simulink model "test_mdl_NI"  (R2018a)
settings: Solver=VariableStepAuto  StartTime=0.0  StopTime=10.0  RelTol=1e-3
(part 12 of 24)

== system test_mdl_NI/Subsystem/IPMA_ADAS/Side_Detect_L_Stat_Ox3A6 ==
  in_port : Inport
  BttLeft_D_RqDrv : Terminator
  BttLeft_D_Stat : Terminator
  CtaAlrtLeft2_D_Stat : Terminator
  CtaAlrtLeft_D_Stat : Terminator
  CtaBrkLeftMsgTxt_B_Rq : Terminator
  CtaLeftBrkDecel_B_Rq : Terminator
  CtaLeftBrkEnbl_B_Rq : Terminator
  CtaLeft_D_Stat : Terminator
  CtaSnsLeft_D_Stat : Terminator
  Side_Detect_L_Illum : Terminator
  SodAlrtLeft_D_Stat : Terminator
  SodDetctLeft_D_Stat : Terminator
  SodLeft_D_Stat : Terminator
  SodSnsLeft_D_Stat : Terminator
  SodWarnLeft_Prd_Rq : Terminator
  bus_selector : BusSelector  OutputSignals=BttLeft_D_RqDrv,BttLeft_D_Stat,CtaAlrtLeft2_D_Stat,CtaAlrtLeft_D_Stat,CtaBrkLeftMsgTxt_B_Rq,CtaLeftBrkDecel_B_Rq,CtaLeftBrkEnbl_B_Rq,CtaLeft_D_Stat,CtaSnsLeft_D_Stat,Side_Detect_L_Illum,SodAlrtLeft_D_Stat,SodDetctLeft_D_Stat,SodLeft_D_Stat,SodSnsLeft_D_Stat,SodWarnLeft_Prd_Rq
  wires:
  in_port/1 -> bus_selector/1  "Side_Detect_L_Stat_Ox3A6"
  bus_selector/1 -> BttLeft_D_RqDrv/1  "<BttLeft_D_RqDrv>"
  bus_selector/2 -> BttLeft_D_Stat/1  "<BttLeft_D_Stat>"
  bus_selector/3 -> CtaAlrtLeft2_D_Stat/1  "<CtaAlrtLeft2_D_Stat>"
  bus_selector/4 -> CtaAlrtLeft_D_Stat/1  "<CtaAlrtLeft_D_Stat>"
  bus_selector/5 -> CtaBrkLeftMsgTxt_B_Rq/1  "<CtaBrkLeftMsgTxt_B_Rq>"
  bus_selector/6 -> CtaLeftBrkDecel_B_Rq/1  "<CtaLeftBrkDecel_B_Rq>"
  bus_selector/7 -> CtaLeftBrkEnbl_B_Rq/1  "<CtaLeftBrkEnbl_B_Rq>"
  bus_selector/8 -> CtaLeft_D_Stat/1  "<CtaLeft_D_Stat>"
  bus_selector/9 -> CtaSnsLeft_D_Stat/1  "<CtaSnsLeft_D_Stat>"
  bus_selector/10 -> Side_Detect_L_Illum/1  "<Side_Detect_L_Illum>"
  bus_selector/11 -> SodAlrtLeft_D_Stat/1  "<SodAlrtLeft_D_Stat>"
  bus_selector/12 -> SodDetctLeft_D_Stat/1  "<SodDetctLeft_D_Stat>"
  bus_selector/13 -> SodLeft_D_Stat/1  "<SodLeft_D_Stat>"
  bus_selector/14 -> SodSnsLeft_D_Stat/1  "<SodSnsLeft_D_Stat>"
  bus_selector/15 -> SodWarnLeft_Prd_Rq/1  "<SodWarnLeft_Prd_Rq>"

== system test_mdl_NI/Subsystem/IPMA_ADAS/Side_Detect_R_Stat_Ox3A7 ==
  in_port : Inport
  BttRight_D_RqDrv : Terminator
  BttRight_D_Stat : Terminator
  CtaAlrtRight2_D_Stat : Terminator
  CtaAlrtRight_D_Stat : Terminator
  CtaBrkRightMsgTxt_B_Rq : Terminator
  CtaRightBrkDecel_B_Rq : Terminator
  CtaRightBrkEnbl_B_Rq : Terminator
  CtaRight_D_Stat : Terminator
  CtaSnsRight_D_Stat : Terminator
  Side_Detect_R_Illum : Terminator
  SodAlrtRight_D_Stat : Terminator
  SodDetctRight_D_Stat : Terminator
  SodRight_D_Stat : Terminator
  SodSnsRight_D_Stat : Terminator
  SodWarnRight_Prd_Rq : Terminator
  bus_selector : BusSelector  OutputSignals=BttRight_D_RqDrv,BttRight_D_Stat,CtaAlrtRight2_D_Stat,CtaAlrtRight_D_Stat,CtaBrkRightMsgTxt_B_Rq,CtaRightBrkDecel_B_Rq,CtaRightBrkEnbl_B_Rq,CtaRight_D_Stat,CtaSnsRight_D_Stat,Side_Detect_R_Illum,SodAlrtRight_D_Stat,SodDetctRight_D_Stat,SodRight_D_Stat,SodSnsRight_D_Stat,SodWarnRight_Prd_Rq
  wires:
  in_port/1 -> bus_selector/1  "Side_Detect_R_Stat_Ox3A7"
  bus_selector/1 -> BttRight_D_RqDrv/1  "<BttRight_D_RqDrv>"
  bus_selector/2 -> BttRight_D_Stat/1  "<BttRight_D_Stat>"
  bus_selector/3 -> CtaAlrtRight2_D_Stat/1  "<CtaAlrtRight2_D_Stat>"
  bus_selector/4 -> CtaAlrtRight_D_Stat/1  "<CtaAlrtRight_D_Stat>"
  bus_selector/5 -> CtaBrkRightMsgTxt_B_Rq/1  "<CtaBrkRightMsgTxt_B_Rq>"
  bus_selector/6 -> CtaRightBrkDecel_B_Rq/1  "<CtaRightBrkDecel_B_Rq>"
  bus_selector/7 -> CtaRightBrkEnbl_B_Rq/1  "<CtaRightBrkEnbl_B_Rq>"
  bus_selector/8 -> CtaRight_D_Stat/1  "<CtaRight_D_Stat>"
  bus_selector/9 -> CtaSnsRight_D_Stat/1  "<CtaSnsRight_D_Stat>"
  bus_selector/10 -> Side_Detect_R_Illum/1  "<Side_Detect_R_Illum>"
  bus_selector/11 -> SodAlrtRight_D_Stat/1  "<SodAlrtRight_D_Stat>"
  bus_selector/12 -> SodDetctRight_D_Stat/1  "<SodDetctRight_D_Stat>"
  bus_selector/13 -> SodRight_D_Stat/1  "<SodRight_D_Stat>"
  bus_selector/14 -> SodSnsRight_D_Stat/1  "<SodSnsRight_D_Stat>"
  bus_selector/15 -> SodWarnRight_Prd_Rq/1  "<SodWarnRight_Prd_Rq>"

== system test_mdl_NI/Subsystem/IPMA_ADAS/Steer_Assist_Data_Ox3D7 ==
  in_port : Inport
  CmbbObjClass_D_Stat : Terminator
  CmbbObjColl_T_Actl : Terminator
  CmbbObjConfdnc_D_Stat : Terminator
  CmbbObjDistLat_L_Actl : Terminator
  CmbbObjDistLong_L_Actl : Terminator
  CmbbObjRelLat_V_Actl : Terminator
  CmbbObjRelLong_V_Actl : Terminator
  EsaEnbl_D2_Rq : Terminator
  bus_selector : BusSelector  OutputSignals=CmbbObjClass_D_Stat,CmbbObjColl_T_Actl,CmbbObjConfdnc_D_Stat,CmbbObjDistLat_L_Actl,CmbbObjDistLong_L_Actl,CmbbObjRelLat_V_Actl,CmbbObjRelLong_V_Actl,EsaEnbl_D2_Rq
  wires:
  in_port/1 -> bus_selector/1  "Steer_Assist_Data_Ox3D7"
  bus_selector/1 -> CmbbObjClass_D_Stat/1  "<CmbbObjClass_D_Stat>"
  bus_selector/2 -> CmbbObjColl_T_Actl/1  "<CmbbObjColl_T_Actl>"
  bus_selector/3 -> CmbbObjConfdnc_D_Stat/1  "<CmbbObjConfdnc_D_Stat>"
  bus_selector/4 -> CmbbObjDistLat_L_Actl/1  "<CmbbObjDistLat_L_Actl>"
  bus_selector/5 -> CmbbObjDistLong_L_Actl/1  "<CmbbObjDistLong_L_Actl>"
  bus_selector/6 -> CmbbObjRelLat_V_Actl/1  "<CmbbObjRelLat_V_Actl>"
  bus_selector/7 -> CmbbObjRelLong_V_Actl/1  "<CmbbObjRelLong_V_Actl>"
  bus_selector/8 -> EsaEnbl_D2_Rq/1  "<EsaEnbl_D2_Rq>"

== system test_mdl_NI/Subsystem/IPMA_ADAS/SuspensionRoad_Data_Ox3D0 ==
  in_port : Inport
  SrpDistLeft_L_Actl : Terminator
  SrpDistRight_L_Actl : Terminator
  SrpEventLeft_D_Stat : Terminator
  SrpEventRight_D_Stat : Terminator
  SrpHghtLeft_L_Actl : Terminator
  SrpHghtRight_L_Actl : Terminator
  SrpSigValid_B_Stat : Terminator
  SuspClkSync_No_Actl : Terminator
  bus_selector : BusSelector  OutputSignals=SrpDistLeft_L_Actl,SrpDistRight_L_Actl,SrpEventLeft_D_Stat,SrpEventRight_D_Stat,SrpHghtLeft_L_Actl,SrpHghtRight_L_Actl,SrpSigValid_B_Stat,SuspClkSync_No_Actl
  wires:
  in_port/1 -> bus_selector/1  "SuspensionRoad_Data_Ox3D0"
  bus_selector/1 -> SrpDistLeft_L_Actl/1  "<SrpDistLeft_L_Actl>"
  bus_selector/2 -> SrpDistRight_L_Actl/1  "<SrpDistRight_L_Actl>"
  bus_selector/3 -> SrpEventLeft_D_Stat/1  "<SrpEventLeft_D_Stat>"
  bus_selector/4 -> SrpEventRight_D_Stat/1  "<SrpEventRight_D_Stat>"
  bus_selector/5 -> SrpHghtLeft_L_Actl/1  "<SrpHghtLeft_L_Actl>"
  bus_selector/6 -> SrpHghtRight_L_Actl/1  "<SrpHghtRight_L_Actl>"
  bus_selector/7 -> SrpSigValid_B_Stat/1  "<SrpSigValid_B_Stat>"
  bus_selector/8 -> SuspClkSync_No_Actl/1  "<SuspClkSync_No_Actl>"

== system test_mdl_NI/Subsystem/IPMA_ADAS/TesterPhysicalResCCM_Ox76C ==
  in_port : Inport
  TesterPhysicalResCCM : Terminator
  bus_selector : BusSelector  OutputSignals=TesterPhysicalResCCM
  wires:
  in_port/1 -> bus_selector/1  "TesterPhysicalResCCM_Ox76C"
  bus_selector/1 -> TesterPhysicalResCCM/1  "<TesterPhysicalResCCM>"

== system test_mdl_NI/Subsystem/IPMA_ADAS/TesterPhysicalResIPMA_Ox70E ==
  in_port : Inport
  TesterPhysicalResIPMA : Terminator
  bus_selector : BusSelector  OutputSignals=TesterPhysicalResIPMA
  wires:
  in_port/1 -> bus_selector/1  "TesterPhysicalResIPMA_Ox70E"
  bus_selector/1 -> TesterPhysicalResIPMA/1  "<TesterPhysicalResIPMA>"

== system test_mdl_NI/Subsystem/IPMA_ADAS/TesterPhysicalResSODCMC_Ox6FA ==
  in_port : Inport
  TesterPhysicalResSODCMC : Terminator
  bus_selector : BusSelector  OutputSignals=TesterPhysicalResSODCMC
  wires:
  in_port/1 -> bus_selector/1  "TesterPhysicalResSODCMC_Ox6FA"
  bus_selector/1 -> TesterPhysicalResSODCMC/1  "<TesterPhysicalResSODCMC>"

== system test_mdl_NI/Subsystem/IPMA_ADAS/TesterPhysicalResSODCMD_Ox6FB ==
  in_port : Inport
  TesterPhysicalResSODCMD : Terminator
  bus_selector : BusSelector  OutputSignals=TesterPhysicalResSODCMD
  wires:
  in_port/1 -> bus_selector/1  "TesterPhysicalResSODCMD_Ox6FB"
  bus_selector/1 -> TesterPhysicalResSODCMD/1  "<TesterPhysicalResSODCMD>"

== system test_mdl_NI/Subsystem/IPMA_ADAS/TesterPhysicalResSODL_Ox7CC ==
  in_port : Inport
  TesterPhysicalResSODL : Terminator
  bus_selector : BusSelector  OutputSignals=TesterPhysicalResSODL
  wires:
  in_port/1 -> bus_selector/1  "TesterPhysicalResSODL_Ox7CC"
  bus_selector/1 -> TesterPhysicalResSODL/1  "<TesterPhysicalResSODL>"

== system test_mdl_NI/Subsystem/IPMA_ADAS/TesterPhysicalResSODR_Ox7CE ==
  in_port : Inport
  TesterPhysicalResSODR : Terminator
  bus_selector : BusSelector  OutputSignals=TesterPhysicalResSODR
  wires:
  in_port/1 -> bus_selector/1  "TesterPhysicalResSODR_Ox7CE"
  bus_selector/1 -> TesterPhysicalResSODR/1  "<TesterPhysicalResSODR>"

== system test_mdl_NI/Subsystem/IPMA_ADAS/Traffic_RecognitnData_Ox3CD ==
  in_port : Inport
  TsrMsgTxt_D_Rq : Terminator
  TsrOswWarnMsgTxt_D_Rq : Terminator
  TsrOvtkMsgTxt2_D_Rq : Terminator
  TsrOvtkMsgTxt_D_Rq : Terminator
  TsrOvtkStatMsgTxt_D_Rq : Terminator
  TsrStatMsgTxt_D_Rq : Terminator
  TsrVLim1MsgTxt_D_Rq : Terminator
  TsrVLim2MsgTxt_D_Rq : Terminator
  TsrVl1PrmntMsgTxt_D_Rq : Terminator
  TsrVl1RstrcMsgTxt2_D_Rq : Terminator
  TsrVl1RstrcMsgTxt_D_Rq : Terminator
  TsrVl1StatMsgTxt_D_Rq : Terminator
  TsrVl2PrmntMsgTxt_D_Rq : Terminator
  TsrVl2RstrcMsgTxt2_D_Rq : Terminator
  TsrVl2RstrcMsgTxt_D_Rq : Terminator
  TsrVl2StatMsgTxt_D_Rq : Terminator
  TsrVlUnitMsgTxt_D_Rq : Terminator
  WwaWarn_B_Rq : Terminator
  bus_selector : BusSelector  OutputSignals=TsrMsgTxt_D_Rq,TsrOswWarnMsgTxt_D_Rq,TsrOvtkMsgTxt2_D_Rq,TsrOvtkMsgTxt_D_Rq,TsrOvtkStatMsgTxt_D_Rq,TsrStatMsgTxt_D_Rq,TsrVLim1MsgTxt_D_Rq,TsrVLim2MsgTxt_D_Rq,TsrVl1PrmntMsgTxt_D_Rq,TsrVl1RstrcMsgTxt2_D_Rq,TsrVl1RstrcMsgTxt_D_Rq,TsrVl1StatMsgTxt_D_Rq,TsrVl2PrmntMsgTxt_D_Rq,TsrVl2RstrcMsgTxt2_D_Rq,TsrVl2RstrcMsgTxt_D_Rq,TsrVl2StatMsgTxt_D_Rq,TsrVlUnitMsgTxt_D_Rq,WwaWarn_B_Rq
  wires:
  in_port/1 -> bus_selector/1  "Traffic_RecognitnData_Ox3CD"
  bus_selector/1 -> TsrMsgTxt_D_Rq/1  "<TsrMsgTxt_D_Rq>"
  bus_selector/2 -> TsrOswWarnMsgTxt_D_Rq/1  "<TsrOswWarnMsgTxt_D_Rq>"
  bus_selector/3 -> TsrOvtkMsgTxt2_D_Rq/1  "<TsrOvtkMsgTxt2_D_Rq>"
  bus_selector/4 -> TsrOvtkMsgTxt_D_Rq/1  "<TsrOvtkMsgTxt_D_Rq>"
  bus_selector/5 -> TsrOvtkStatMsgTxt_D_Rq/1  "<TsrOvtkStatMsgTxt_D_Rq>"
  bus_selector/6 -> TsrStatMsgTxt_D_Rq/1  "<TsrStatMsgTxt_D_Rq>"
  bus_selector/7 -> TsrVLim1MsgTxt_D_Rq/1  "<TsrVLim1MsgTxt_D_Rq>"
  bus_selector/8 -> TsrVLim2MsgTxt_D_Rq/1  "<TsrVLim2MsgTxt_D_Rq>"
  bus_selector/9 -> TsrVl1PrmntMsgTxt_D_Rq/1  "<TsrVl1PrmntMsgTxt_D_Rq>"
  bus_selector/10 -> TsrVl1RstrcMsgTxt2_D_Rq/1  "<TsrVl1RstrcMsgTxt2_D_Rq>"
  bus_selector/11 -> TsrVl1RstrcMsgTxt_D_Rq/1  "<TsrVl1RstrcMsgTxt_D_Rq>"
  bus_selector/12 -> TsrVl1StatMsgTxt_D_Rq/1  "<TsrVl1StatMsgTxt_D_Rq>"
  bus_selector/13 -> TsrVl2PrmntMsgTxt_D_Rq/1  "<TsrVl2PrmntMsgTxt_D_Rq>"
  bus_selector/14 -> TsrVl2RstrcMsgTxt2_D_Rq/1  "<TsrVl2RstrcMsgTxt2_D_Rq>"
  bus_selector/15 -> TsrVl2RstrcMsgTxt_D_Rq/1  "<TsrVl2RstrcMsgTxt_D_Rq>"
  bus_selector/16 -> TsrVl2StatMsgTxt_D_Rq/1  "<TsrVl2StatMsgTxt_D_Rq>"
  bus_selector/17 -> TsrVlUnitMsgTxt_D_Rq/1  "<TsrVlUnitMsgTxt_D_Rq>"
  bus_selector/18 -> WwaWarn_B_Rq/1  "<WwaWarn_B_Rq>"

== system test_mdl_NI/Subsystem/IPMA_ADAS/TrailerAid_Stat3_Ox459 ==
  in_port : Inport
  HitchToTrlrAxle_L_Calc2 : Terminator
  HitchToVehAxle_L_Calc : Terminator
  TrlrAidTrgtId_No_Actl : Terminator
  TrlrAid_An3_Actl : Terminator
  TrlrAid_AnRate2_Actl : Terminator
  TrlrAid_D2_Stat : Terminator
  TrlrAnCalib_B_Complt : Terminator
  TrlrAnOffstDir_D_Calc : Terminator
  TrlrAnOffst_An_Calc : Terminator
  TrlrRvrse_D_Stat : Terminator
  TrlrTrgtAcquire_D_Stat : Terminator
  bus_selector : BusSelector  OutputSignals=HitchToTrlrAxle_L_Calc2,HitchToVehAxle_L_Calc,TrlrAidTrgtId_No_Actl,TrlrAid_An3_Actl,TrlrAid_AnRate2_Actl,TrlrAid_D2_Stat,TrlrAnCalib_B_Complt,TrlrAnOffstDir_D_Calc,TrlrAnOffst_An_Calc,TrlrRvrse_D_Stat,TrlrTrgtAcquire_D_Stat
  wires:
  in_port/1 -> bus_selector/1  "TrailerAid_Stat3_Ox459"
  bus_selector/1 -> HitchToTrlrAxle_L_Calc2/1  "<HitchToTrlrAxle_L_Calc2>"
  bus_selector/2 -> HitchToVehAxle_L_Calc/1  "<HitchToVehAxle_L_Calc>"
  bus_selector/3 -> TrlrAidTrgtId_No_Actl/1  "<TrlrAidTrgtId_No_Actl>"
  bus_selector/4 -> TrlrAid_An3_Actl/1  "<TrlrAid_An3_Actl>"
  bus_selector/5 -> TrlrAid_AnRate2_Actl/1  "<TrlrAid_AnRate2_Actl>"
  bus_selector/6 -> TrlrAid_D2_Stat/1  "<TrlrAid_D2_Stat>"
  bus_selector/7 -> TrlrAnCalib_B_Complt/1  "<TrlrAnCalib_B_Complt>"
  bus_selector/8 -> TrlrAnOffstDir_D_Calc/1  "<TrlrAnOffstDir_D_Calc>"
  bus_selector/9 -> TrlrAnOffst_An_Calc/1  "<TrlrAnOffst_An_Calc>"
  bus_selector/10 -> TrlrRvrse_D_Stat/1  "<TrlrRvrse_D_Stat>"
  bus_selector/11 -> TrlrTrgtAcquire_D_Stat/1  "<TrlrTrgtAcquire_D_Stat>"

== system test_mdl_NI/Subsystem/PCM/DCACA_Data4_Ox36E ==
  in_port : Inport
  DcacElPw_D_Stat : Terminator
  DcacEngOnMsgTxt_D_Rq : Terminator
  DcacFaltMsgTxt_D_Rq : Terminator
  DcacGfciTest_B_Rq : Terminator
  DcacHw_D_Confg : Terminator
  DcacLedCtl_D_Rq : Terminator
  DcacLoFuelMsgTxt_D_Rq : Terminator
  DcacOn_B_Rq : Terminator
  DcacOut1_Pw_Dsply : Terminator
  DcacOut2_Pw_Dsply : Terminator
  DcacOut_Pw_DsplyMx : Terminator
  DcacSys_B_Falt : Terminator
  PwBedPnlEnbl_B_Rq : Terminator
  bus_selector : BusSelector  OutputSignals=DcacElPw_D_Stat,DcacEngOnMsgTxt_D_Rq,DcacFaltMsgTxt_D_Rq,DcacGfciTest_B_Rq,DcacHw_D_Confg,DcacLedCtl_D_Rq,DcacLoFuelMsgTxt_D_Rq,DcacOn_B_Rq,DcacOut1_Pw_Dsply,DcacOut2_Pw_Dsply,DcacOut_Pw_DsplyMx,DcacSys_B_Falt,PwBedPnlEnbl_B_Rq
  wires:
  in_port/1 -> bus_selector/1  "DCACA_Data4_Ox36E"
  bus_selector/1 -> DcacElPw_D_Stat/1  "<DcacElPw_D_Stat>"
  bus_selector/2 -> DcacEngOnMsgTxt_D_Rq/1  "<DcacEngOnMsgTxt_D_Rq>"
  bus_selector/3 -> DcacFaltMsgTxt_D_Rq/1  "<DcacFaltMsgTxt_D_Rq>"
  bus_selector/4 -> DcacGfciTest_B_Rq/1  "<DcacGfciTest_B_Rq>"
  bus_selector/5 -> DcacHw_D_Confg/1  "<DcacHw_D_Confg>"
  bus_selector/6 -> DcacLedCtl_D_Rq/1  "<DcacLedCtl_D_Rq>"
  bus_selector/7 -> DcacLoFuelMsgTxt_D_Rq/1  "<DcacLoFuelMsgTxt_D_Rq>"
  bus_selector/8 -> DcacOn_B_Rq/1  "<DcacOn_B_Rq>"
  bus_selector/9 -> DcacOut1_Pw_Dsply/1  "<DcacOut1_Pw_Dsply>"
  bus_selector/10 -> DcacOut2_Pw_Dsply/1  "<DcacOut2_Pw_Dsply>"
  bus_selector/11 -> DcacOut_Pw_DsplyMx/1  "<DcacOut_Pw_DsplyMx>"
  bus_selector/12 -> DcacSys_B_Falt/1  "<DcacSys_B_Falt>"
  bus_selector/13 -> PwBedPnlEnbl_B_Rq/1  "<PwBedPnlEnbl_B_Rq>"

== system test_mdl_NI/Subsystem/PCM/EngBrakeData_Ox165 ==
  in_port : Inport
  AccEngStat_D_Actl : Terminator
  AccStopMde_D_Rq : Terminator
  BPedDrvAppl_D_QF : Terminator
  BpedDrvAppl_D_Actl : Terminator
  CcMde_D_Actl : Terminator
  CcOvrrdActv_B_Actl : Terminator
  CcStat_D_Actl : Terminator
  CmbbDeny_B_ActlPrpl : Terminator
  CmbbEngTqMn_B_Actl : Terminator
  EngAout_N_MnAllw : Terminator
  PrplTqMnSat_B_Actl : Terminator
  Veh_V_DsplyCcSet : Terminator
  bus_selector : BusSelector  OutputSignals=AccEngStat_D_Actl,AccStopMde_D_Rq,BPedDrvAppl_D_QF,BpedDrvAppl_D_Actl,CcMde_D_Actl,CcOvrrdActv_B_Actl,CcStat_D_Actl,CmbbDeny_B_ActlPrpl,CmbbEngTqMn_B_Actl,EngAout_N_MnAllw,PrplTqMnSat_B_Actl,Veh_V_DsplyCcSet
  wires:
  in_port/1 -> bus_selector/1  "EngBrakeData_Ox165"
  bus_selector/1 -> AccEngStat_D_Actl/1  "<AccEngStat_D_Actl>"
  bus_selector/2 -> AccStopMde_D_Rq/1  "<AccStopMde_D_Rq>"
  bus_selector/3 -> BPedDrvAppl_D_QF/1  "<BPedDrvAppl_D_QF>"
  bus_selector/4 -> BpedDrvAppl_D_Actl/1  "<BpedDrvAppl_D_Actl>"
  bus_selector/5 -> CcMde_D_Actl/1  "<CcMde_D_Actl>"
  bus_selector/6 -> CcOvrrdActv_B_Actl/1  "<CcOvrrdActv_B_Actl>"
  bus_selector/7 -> CcStat_D_Actl/1  "<CcStat_D_Actl>"
  bus_selector/8 -> CmbbDeny_B_ActlPrpl/1  "<CmbbDeny_B_ActlPrpl>"
  bus_selector/9 -> CmbbEngTqMn_B_Actl/1  "<CmbbEngTqMn_B_Actl>"
  bus_selector/10 -> EngAout_N_MnAllw/1  "<EngAout_N_MnAllw>"
  bus_selector/11 -> PrplTqMnSat_B_Actl/1  "<PrplTqMnSat_B_Actl>"
  bus_selector/12 -> Veh_V_DsplyCcSet/1  "<Veh_V_DsplyCcSet>"

== system test_mdl_NI/Subsystem/PCM/EngVehicleSpThrottle2_Ox202 ==
  in_port : Inport
  GearRvrse_D_Actl : Terminator
  StrtrMtrCtlMsgTxt_D2_Rq : Terminator
  StrtrMtrCtlMsgTxt_D_Rq : Terminator
  StrtrMtrDlyStrt_B_Stat : Terminator
  VehVActlEng_D_Qf : Terminator
  VehVActlEng_No_Cnt : Terminator
  VehVActlEng_No_Cs : Terminator
  VehVTrlrAid_B_Avail : Terminator
  Veh_V_ActlEng : Terminator
  Veh_V_RqCcSet : Terminator
  bus_selector : BusSelector  OutputSignals=GearRvrse_D_Actl,StrtrMtrCtlMsgTxt_D2_Rq,StrtrMtrCtlMsgTxt_D_Rq,StrtrMtrDlyStrt_B_Stat,VehVActlEng_D_Qf,VehVActlEng_No_Cnt,VehVActlEng_No_Cs,VehVTrlrAid_B_Avail,Veh_V_ActlEng,Veh_V_RqCcSet
  wires:
  in_port/1 -> bus_selector/1  "EngVehicleSpThrottle2_Ox202"
  bus_selector/1 -> GearRvrse_D_Actl/1  "<GearRvrse_D_Actl>"
  bus_selector/2 -> StrtrMtrCtlMsgTxt_D2_Rq/1  "<StrtrMtrCtlMsgTxt_D2_Rq>"
  bus_selector/3 -> StrtrMtrCtlMsgTxt_D_Rq/1  "<StrtrMtrCtlMsgTxt_D_Rq>"
  bus_selector/4 -> StrtrMtrDlyStrt_B_Stat/1  "<StrtrMtrDlyStrt_B_Stat>"
  bus_selector/5 -> VehVActlEng_D_Qf/1  "<VehVActlEng_D_Qf>"
  bus_selector/6 -> VehVActlEng_No_Cnt/1  "<VehVActlEng_No_Cnt>"
  bus_selector/7 -> VehVActlEng_No_Cs/1  "<VehVActlEng_No_Cs>"
  bus_selector/8 -> VehVTrlrAid_B_Avail/1  "<VehVTrlrAid_B_Avail>"
  bus_selector/9 -> Veh_V_ActlEng/1  "<Veh_V_ActlEng>"
  bus_selector/10 -> Veh_V_RqCcSet/1  "<Veh_V_RqCcSet>"

== system test_mdl_NI/Subsystem/PCM/EngVehicleSpThrottle_Ox204 ==
  in_port : Inport
  ApedPosPcActl_D_Qf : Terminator
  ApedPosPcActl_No_Cnt : Terminator
  ApedPosPcActl_No_Cs : Terminator
  ApedPos_PcRate_ActlArb : Terminator
  ApedPos_Pc_ActlArb : Terminator
  EngAout3_N_Actl : Terminator
  EngAoutNActl_D_QF : Terminator
  EngAout_N_Actl : Terminator
  bus_selector : BusSelector  OutputSignals=ApedPosPcActl_D_Qf,ApedPosPcActl_No_Cnt,ApedPosPcActl_No_Cs,ApedPos_PcRate_ActlArb,ApedPos_Pc_ActlArb,EngAout3_N_Actl,EngAoutNActl_D_QF,EngAout_N_Actl
  wires:
  in_port/1 -> bus_selector/1  "EngVehicleSpThrottle_Ox204"
  bus_selector/1 -> ApedPosPcActl_D_Qf/1  "<ApedPosPcActl_D_Qf>"
  bus_selector/2 -> ApedPosPcActl_No_Cnt/1  "<ApedPosPcActl_No_Cnt>"
  bus_selector/3 -> ApedPosPcActl_No_Cs/1  "<ApedPosPcActl_No_Cs>"
  bus_selector/4 -> ApedPos_PcRate_ActlArb/1  "<ApedPos_PcRate_ActlArb>"
  bus_selector/5 -> ApedPos_Pc_ActlArb/1  "<ApedPos_Pc_ActlArb>"
  bus_selector/6 -> EngAout3_N_Actl/1  "<EngAout3_N_Actl>"
  bus_selector/7 -> EngAoutNActl_D_QF/1  "<EngAoutNActl_D_QF>"
  bus_selector/8 -> EngAout_N_Actl/1  "<EngAout_N_Actl>"

== system test_mdl_NI/Subsystem/PCM/EngineClimateData_Ox178 ==
  in_port : Inport
  AirAmbTe_D_Qf : Terminator
  AirAmb_P_Actl : Terminator
  AirAmb_Te_Actl : Terminator
  AirAmb_Te_ActlFilt : Terminator
  AslChime_B_Rq : Terminator
  AslIconDsply_D_Rq : Terminator
  DynoMde_B_Cmd : Terminator
  EcssLamp_D_RqDsply : Terminator
  EngAout_Aa_Actl : Terminator
  GasPrtc_D_RqDsply : Terminator
  HvacHtrCore2_Te_Actl : Terminator
  bus_selector : BusSelector  OutputSignals=AirAmbTe_D_Qf,AirAmb_P_Actl,AirAmb_Te_Actl,AirAmb_Te_ActlFilt,AslChime_B_Rq,AslIconDsply_D_Rq,DynoMde_B_Cmd,EcssLamp_D_RqDsply,EngAout_Aa_Actl,GasPrtc_D_RqDsply,HvacHtrCore2_Te_Actl
  wires:
  in_port/1 -> bus_selector/1  "EngineClimateData_Ox178"
  bus_selector/1 -> AirAmbTe_D_Qf/1  "<AirAmbTe_D_Qf>"
  bus_selector/2 -> AirAmb_P_Actl/1  "<AirAmb_P_Actl>"
  bus_selector/3 -> AirAmb_Te_Actl/1  "<AirAmb_Te_Actl>"
  bus_selector/4 -> AirAmb_Te_ActlFilt/1  "<AirAmb_Te_ActlFilt>"
  bus_selector/5 -> AslChime_B_Rq/1  "<AslChime_B_Rq>"
  bus_selector/6 -> AslIconDsply_D_Rq/1  "<AslIconDsply_D_Rq>"
  bus_selector/7 -> DynoMde_B_Cmd/1  "<DynoMde_B_Cmd>"
  bus_selector/8 -> EcssLamp_D_RqDsply/1  "<EcssLamp_D_RqDsply>"
  bus_selector/9 -> EngAout_Aa_Actl/1  "<EngAout_Aa_Actl>"
  bus_selector/10 -> GasPrtc_D_RqDsply/1  "<GasPrtc_D_RqDsply>"
  bus_selector/11 -> HvacHtrCore2_Te_Actl/1  "<HvacHtrCore2_Te_Actl>"

== system test_mdl_NI/Subsystem/PCM/EngineData_16_Ox17C ==
  in_port : Inport
  EngAout_N_MxAllw : Terminator
  EngExhBrkAutoLamp_B_Rq : Terminator
  EngExhBrkMde_D_Actl : Terminator
  EngExhBrkOnLamp_B_Rq : Terminator
  EngOilLvlWarn_D_Rq1 : Terminator
  bus_selector : BusSelector  OutputSignals=EngAout_N_MxAllw,EngExhBrkAutoLamp_B_Rq,EngExhBrkMde_D_Actl,EngExhBrkOnLamp_B_Rq,EngOilLvlWarn_D_Rq1
  wires:
  in_port/1 -> bus_selector/1  "EngineData_16_Ox17C"
  bus_selector/1 -> EngAout_N_MxAllw/1  "<EngAout_N_MxAllw>"
  bus_selector/2 -> EngExhBrkAutoLamp_B_Rq/1  "<EngExhBrkAutoLamp_B_Rq>"
  bus_selector/3 -> EngExhBrkMde_D_Actl/1  "<EngExhBrkMde_D_Actl>"
  bus_selector/4 -> EngExhBrkOnLamp_B_Rq/1  "<EngExhBrkOnLamp_B_Rq>"
  bus_selector/5 -> EngOilLvlWarn_D_Rq1/1  "<EngOilLvlWarn_D_Rq1>"

== system test_mdl_NI/Subsystem/PCM/EngineData_1_Ox171 ==
  in_port : Inport
  SeatWorkSrfc_B_Falt : Terminator
  TrnIpcDsplyGear_D_Actl : Terminator
  TrnIpcDsplyGear_D_Stat : Terminator
  TrnIpcDsplyMde_D_Actl : Terminator
  TrnIpcDsplyMde_D_Stat : Terminator
  TrnIpcDsplyRng2_D_Actl : Terminator
  TrnIpcDsplyRng_D_Stat : Terminator
  bus_selector : BusSelector  OutputSignals=SeatWorkSrfc_B_Falt,TrnIpcDsplyGear_D_Actl,TrnIpcDsplyGear_D_Stat,TrnIpcDsplyMde_D_Actl,TrnIpcDsplyMde_D_Stat,TrnIpcDsplyRng2_D_Actl,TrnIpcDsplyRng_D_Stat
  wires:
  in_port/1 -> bus_selector/1  "EngineData_1_Ox171"
  bus_selector/1 -> SeatWorkSrfc_B_Falt/1  "<SeatWorkSrfc_B_Falt>"
  bus_selector/2 -> TrnIpcDsplyGear_D_Actl/1  "<TrnIpcDsplyGear_D_Actl>"
  bus_selector/3 -> TrnIpcDsplyGear_D_Stat/1  "<TrnIpcDsplyGear_D_Stat>"
  bus_selector/4 -> TrnIpcDsplyMde_D_Actl/1  "<TrnIpcDsplyMde_D_Actl>"
  bus_selector/5 -> TrnIpcDsplyMde_D_Stat/1  "<TrnIpcDsplyMde_D_Stat>"
  bus_selector/6 -> TrnIpcDsplyRng2_D_Actl/1  "<TrnIpcDsplyRng2_D_Actl>"
  bus_selector/7 -> TrnIpcDsplyRng_D_Stat/1  "<TrnIpcDsplyRng_D_Stat>"

== system test_mdl_NI/Subsystem/PCM/EngineData_6_Ox156 ==
  in_port : Inport
  EngClntTe_D_Qf : Terminator
  EngClnt_Te_Actl : Terminator
  EngGoutLss_Tq_Est : Terminator
  EngOil_Te_Actl : Terminator
  EngOvrhtMitgActv_D_Ind : Terminator
  bus_selector : BusSelector  OutputSignals=EngClntTe_D_Qf,EngClnt_Te_Actl,EngGoutLss_Tq_Est,EngOil_Te_Actl,EngOvrhtMitgActv_D_Ind
  wires:
  in_port/1 -> bus_selector/1  "EngineData_6_Ox156"
  bus_selector/1 -> EngClntTe_D_Qf/1  "<EngClntTe_D_Qf>"
  bus_selector/2 -> EngClnt_Te_Actl/1  "<EngClnt_Te_Actl>"
  bus_selector/3 -> EngGoutLss_Tq_Est/1  "<EngGoutLss_Tq_Est>"
  bus_selector/4 -> EngOil_Te_Actl/1  "<EngOil_Te_Actl>"
  bus_selector/5 -> EngOvrhtMitgActv_D_Ind/1  "<EngOvrhtMitgActv_D_Ind>"

== system test_mdl_NI/Subsystem/PCM/EngineData_7_Ox179 ==
  in_port : Inport
  AirCondClutch_B_Stats : Terminator
  AirCondRec_B_Rq : Terminator
  EngOilLife_Pc_Actl : Terminator
  EngSrvcRqd_B_Rq : Terminator
  FuelFillInlet_B_Dsply : Terminator
  FuelFilterLamp_B_Dsply : Terminator
  FuelFlw_Vl_Dsply : Terminator
  HvacAirFullOut_B_Rq : Terminator
  OdoCount : Terminator
  bus_selector : BusSelector  OutputSignals=AirCondClutch_B_Stats,AirCondRec_B_Rq,EngOilLife_Pc_Actl,EngSrvcRqd_B_Rq,FuelFillInlet_B_Dsply,FuelFilterLamp_B_Dsply,FuelFlw_Vl_Dsply,HvacAirFullOut_B_Rq,OdoCount
  wires:
  in_port/1 -> bus_selector/1  "EngineData_7_Ox179"
  bus_selector/1 -> AirCondClutch_B_Stats/1  "<AirCondClutch_B_Stats>"
  bus_selector/2 -> AirCondRec_B_Rq/1  "<AirCondRec_B_Rq>"
  bus_selector/3 -> EngOilLife_Pc_Actl/1  "<EngOilLife_Pc_Actl>"
  bus_selector/4 -> EngSrvcRqd_B_Rq/1  "<EngSrvcRqd_B_Rq>"
  bus_selector/5 -> FuelFillInlet_B_Dsply/1  "<FuelFillInlet_B_Dsply>"
  bus_selector/6 -> FuelFilterLamp_B_Dsply/1  "<FuelFilterLamp_B_Dsply>"
  bus_selector/7 -> FuelFlw_Vl_Dsply/1  "<FuelFlw_Vl_Dsply>"
  bus_selector/8 -> HvacAirFullOut_B_Rq/1  "<HvacAirFullOut_B_Rq>"
  bus_selector/9 -> OdoCount/1  "<OdoCount>"

== system test_mdl_NI/Subsystem/PCM/Engine_Clutch_Data_Ox42F ==
  in_port : Inport
  CluPdlPosPcMeas_D_Qf : Terminator
  CluPdlPos_Pc_Meas : Terminator
  CluPdl_PcRate_Actl : Terminator
  EngAoutIdl_N_Ntrl : Terminator
  EngAout_N_Dsply : Terminator
  bus_selector : BusSelector  OutputSignals=CluPdlPosPcMeas_D_Qf,CluPdlPos_Pc_Meas,CluPdl_PcRate_Actl,EngAoutIdl_N_Ntrl,EngAout_N_Dsply
  wires:
  in_port/1 -> bus_selector/1  "Engine_Clutch_Data_Ox42F"
  bus_selector/1 -> CluPdlPosPcMeas_D_Qf/1  "<CluPdlPosPcMeas_D_Qf>"
  bus_selector/2 -> CluPdlPos_Pc_Meas/1  "<CluPdlPos_Pc_Meas>"
  bus_selector/3 -> CluPdl_PcRate_Actl/1  "<CluPdl_PcRate_Actl>"
  bus_selector/4 -> EngAoutIdl_N_Ntrl/1  "<EngAoutIdl_N_Ntrl>"
  bus_selector/5 -> EngAout_N_Dsply/1  "<EngAout_N_Dsply>"

== system test_mdl_NI/Subsystem/PCM/Gear_Shift_by_Wire_3_Ox5C ==
  in_port : Inport
  GearSelLck_D_Rq : Terminator
  PrkBrkActv_D_RqTrnGear : Terminator
  TrnCmdCnt_B_Actl : Terminator
  TrnCmdState_B_Actl : Terminator
  TrnDtpCmd_D_Actl : Terminator
  TrnGearCmd_No_Cnt : Terminator
  TrnGearCmd_No_Cs : Terminator
  TrnGearCmd_Pc_ActlPt : Terminator
  TrnGearMsgTxt_D_Rq : Terminator
  TrnGearNtmAllow_B_Stat : Terminator
  TrnGear_D_RqPt : Terminator
  TrnLvrV_D_Rq : Terminator
  TrnNtrlTowCmd_D_Actl : Terminator
  TrnSbwSysHlth_D_Actl : Terminator
  TrnValidGear_D_Cnfm : Terminator
  bus_selector : BusSelector  OutputSignals=GearSelLck_D_Rq,PrkBrkActv_D_RqTrnGear,TrnCmdCnt_B_Actl,TrnCmdState_B_Actl,TrnDtpCmd_D_Actl,TrnGearCmd_No_Cnt,TrnGearCmd_No_Cs,TrnGearCmd_Pc_ActlPt,TrnGearMsgTxt_D_Rq,TrnGearNtmAllow_B_Stat,TrnGear_D_RqPt,TrnLvrV_D_Rq,TrnNtrlTowCmd_D_Actl,TrnSbwSysHlth_D_Actl,TrnValidGear_D_Cnfm
  wires:
  in_port/1 -> bus_selector/1  "Gear_Shift_by_Wire_3_Ox5C"
  bus_selector/1 -> GearSelLck_D_Rq/1  "<GearSelLck_D_Rq>"
  bus_selector/2 -> PrkBrkActv_D_RqTrnGear/1  "<PrkBrkActv_D_RqTrnGear>"
  bus_selector/3 -> TrnCmdCnt_B_Actl/1  "<TrnCmdCnt_B_Actl>"
  bus_selector/4 -> TrnCmdState_B_Actl/1  "<TrnCmdState_B_Actl>"
  bus_selector/5 -> TrnDtpCmd_D_Actl/1  "<TrnDtpCmd_D_Actl>"
  bus_selector/6 -> TrnGearCmd_No_Cnt/1  "<TrnGearCmd_No_Cnt>"
  bus_selector/7 -> TrnGearCmd_No_Cs/1  "<TrnGearCmd_No_Cs>"
  bus_selector/8 -> TrnGearCmd_Pc_ActlPt/1  "<TrnGearCmd_Pc_ActlPt>"
  bus_selector/9 -> TrnGearMsgTxt_D_Rq/1  "<TrnGearMsgTxt_D_Rq>"
  bus_selector/10 -> TrnGearNtmAllow_B_Stat/1  "<TrnGearNtmAllow_B_Stat>"
  bus_selector/11 -> TrnGear_D_RqPt/1  "<TrnGear_D_RqPt>"
  bus_selector/12 -> TrnLvrV_D_Rq/1  "<TrnLvrV_D_Rq>"
  bus_selector/13 -> TrnNtrlTowCmd_D_Actl/1  "<TrnNtrlTowCmd_D_Actl>"
  bus_selector/14 -> TrnSbwSysHlth_D_Actl/1  "<TrnSbwSysHlth_D_Actl>"
  bus_selector/15 -> TrnValidGear_D_Cnfm/1  "<TrnValidGear_D_Cnfm>"

== system test_mdl_NI/Subsystem/PCM/Global_PATS_TargetInfo_Ox47 ==
  in_port : Inport
  bus_selector : BusSelector  OutputSignals=immoTarget1Cmd,immoTarget1Data,immoTarget1Status
  immoTarget1Cmd : Terminator
  immoTarget1Data : Terminator
  immoTarget1Status : Terminator
  wires:
  in_port/1 -> bus_selector/1  "Global_PATS_TargetInfo_Ox47"
  bus_selector/1 -> immoTarget1Cmd/1  "<immoTarget1Cmd>"
  bus_selector/2 -> immoTarget1Data/1  "<immoTarget1Data>"
  bus_selector/3 -> immoTarget1Status/1  "<immoTarget1Status>"

== system test_mdl_NI/Subsystem/PCM/Low_Voltage_Power_Data_FD1_Ox43D ==
  in_port : Inport
  PwSrcULoComm_B_Falt : Terminator
  PwSrcULoDcnnt_B_Stat : Terminator
  PwSrcULoFalt_D_Stat : Terminator
  PwSrcULoOvrTe_B_Actl : Terminator
  PwSrcULo_I_Actl : Terminator
  PwSrcULo_I_Mx : Terminator
  PwSrcULo_Pc_Mx : Terminator
  ULoRgenTestMde_B_Stat : Terminator
  bus_selector : BusSelector  OutputSignals=PwSrcULoComm_B_Falt,PwSrcULoDcnnt_B_Stat,PwSrcULoFalt_D_Stat,PwSrcULoOvrTe_B_Actl,PwSrcULo_I_Actl,PwSrcULo_I_Mx,PwSrcULo_Pc_Mx,ULoRgenTestMde_B_Stat
  wires:
  in_port/1 -> bus_selector/1  "Low_Voltage_Power_Data_FD1_Ox43D"
  bus_selector/1 -> PwSrcULoComm_B_Falt/1  "<PwSrcULoComm_B_Falt>"
  bus_selector/2 -> PwSrcULoDcnnt_B_Stat/1  "<PwSrcULoDcnnt_B_Stat>"
  bus_selector/3 -> PwSrcULoFalt_D_Stat/1  "<PwSrcULoFalt_D_Stat>"
  bus_selector/4 -> PwSrcULoOvrTe_B_Actl/1  "<PwSrcULoOvrTe_B_Actl>"
  bus_selector/5 -> PwSrcULo_I_Actl/1  "<PwSrcULo_I_Actl>"
  bus_selector/6 -> PwSrcULo_I_Mx/1  "<PwSrcULo_I_Mx>"
  bus_selector/7 -> PwSrcULo_Pc_Mx/1  "<PwSrcULo_Pc_Mx>"
  bus_selector/8 -> ULoRgenTestMde_B_Stat/1  "<ULoRgenTestMde_B_Stat>"

== system test_mdl_NI/Subsystem/PCM/OTAPhysPCMtoGWM_ECG_Ox1B936010 ==
  in_port : Inport
  OTAPhysPCMtoGWM_ECG : Terminator
  bus_selector : BusSelector  OutputSignals=OTAPhysPCMtoGWM_ECG
  wires:
  in_port/1 -> bus_selector/1  "OTAPhysPCMtoGWM_ECG_Ox1B936010"
  bus_selector/1 -> OTAPhysPCMtoGWM_ECG/1  "<OTAPhysPCMtoGWM_ECG>"

== system test_mdl_NI/Subsystem/PCM/PARSEDPhysPCMtoGWM_ECG_Ox1BA36010 ==
  in_port : Inport
  PARSEDPhysPCMtoGWM_ECG : Terminator
  bus_selector : BusSelector  OutputSignals=PARSEDPhysPCMtoGWM_ECG
  wires:
  in_port/1 -> bus_selector/1  "PARSEDPhysPCMtoGWM_ECG_Ox1BA36010"
  bus_selector/1 -> PARSEDPhysPCMtoGWM_ECG/1  "<PARSEDPhysPCMtoGWM_ECG>"

== system test_mdl_NI/Subsystem/PCM/PARSEDPushPCMtoGWM_ECG_Ox1BB36010 ==
  in_port : Inport
  PARSEDPushPCMtoGWM_ECG : Terminator
  bus_selector : BusSelector  OutputSignals=PARSEDPushPCMtoGWM_ECG
  wires:
  in_port/1 -> bus_selector/1  "PARSEDPushPCMtoGWM_ECG_Ox1BB36010"
  bus_selector/1 -> PARSEDPushPCMtoGWM_ECG/1  "<PARSEDPushPCMtoGWM_ECG>"

== system test_mdl_NI/Subsystem/PCM/PCM_AutoSar_NetworkMgmt_Ox595 ==
  in_port : Inport
  PCM_AutoSarNMControl : Terminator
  PCM_AutoSarNMNodeId : Terminator
  PCM_AutoSarNMReserved{1..4} (4 alike) : Terminator
  PCM_GWNMProxy : Terminator
  PCM_GWOnBoardTester : Terminator
  bus_selector : BusSelector  OutputSignals=PCM_AutoSarNMControl,PCM_AutoSarNMNodeId,PCM_AutoSarNMReserved1,PCM_AutoSarNMReserved2,PCM_AutoSarNMReserved3,PCM_AutoSarNMReserved4,PCM_GWNMProxy,PCM_GWOnBoardTester
  wires:
  in_port/1 -> bus_selector/1  "PCM_AutoSar_NetworkMgmt_Ox595"
  bus_selector/1 -> PCM_AutoSarNMControl/1  "<PCM_AutoSarNMControl>"
  bus_selector/2 -> PCM_AutoSarNMNodeId/1  "<PCM_AutoSarNMNodeId>"
  bus_selector/3 -> PCM_AutoSarNMReserved1/1  "<PCM_AutoSarNMReserved1>"
  bus_selector/4 -> PCM_AutoSarNMReserved2/1  "<PCM_AutoSarNMReserved2>"
  bus_selector/5 -> PCM_AutoSarNMReserved3/1  "<PCM_AutoSarNMReserved3>"
  bus_selector/6 -> PCM_AutoSarNMReserved4/1  "<PCM_AutoSarNMReserved4>"
  bus_selector/7 -> PCM_GWNMProxy/1  "<PCM_GWNMProxy>"
  bus_selector/8 -> PCM_GWOnBoardTester/1  "<PCM_GWOnBoardTester>"

== system test_mdl_NI/Subsystem/PCM/PCM_Rapid_Data_Response_1_Ox6A0 ==
  in_port : Inport
  UUDTPCMResponse1 : Terminator
  bus_selector : BusSelector  OutputSignals=UUDTPCMResponse1
  wires:
  in_port/1 -> bus_selector/1  "PCM_Rapid_Data_Response_1_Ox6A0"
  bus_selector/1 -> UUDTPCMResponse1/1  "<UUDTPCMResponse1>"

== system test_mdl_NI/Subsystem/PCM/PCM_Rapid_Data_Response_2_Ox6A1 ==
  in_port : Inport
  UUDTPCMResponse2 : Terminator
  bus_selector : BusSelector  OutputSignals=UUDTPCMResponse2
  wires:
  in_port/1 -> bus_selector/1  "PCM_Rapid_Data_Response_2_Ox6A1"
  bus_selector/1 -> UUDTPCMResponse2/1  "<UUDTPCMResponse2>"

== system test_mdl_NI/Subsystem/PCM/PowertrainData_10_Ox176 ==
  in_port : Inport
  GearEngag_D_Actl : Terminator
  GearLvr_D_ActlDrv : Terminator
  GearPos_D_Actl : Terminator
  GearPos_D_Trg : Terminator
  GearPos_No_Cnt : Terminator
  GearPos_No_Cs : Terminator
  TrnIgnOffDly_T_Rq : Terminator
  TrnPrkSys_D_Actl : Terminator
  TrnRng_D_Rq : Terminator
  bus_selector : BusSelector  OutputSignals=GearEngag_D_Actl,GearLvr_D_ActlDrv,GearPos_D_Actl,GearPos_D_Trg,GearPos_No_Cnt,GearPos_No_Cs,TrnIgnOffDly_T_Rq,TrnPrkSys_D_Actl,TrnRng_D_Rq
  wires:
  in_port/1 -> bus_selector/1  "PowertrainData_10_Ox176"
  bus_selector/1 -> GearEngag_D_Actl/1  "<GearEngag_D_Actl>"
  bus_selector/2 -> GearLvr_D_ActlDrv/1  "<GearLvr_D_ActlDrv>"
  bus_selector/3 -> GearPos_D_Actl/1  "<GearPos_D_Actl>"
  bus_selector/4 -> GearPos_D_Trg/1  "<GearPos_D_Trg>"
  bus_selector/5 -> GearPos_No_Cnt/1  "<GearPos_No_Cnt>"
  bus_selector/6 -> GearPos_No_Cs/1  "<GearPos_No_Cs>"
  bus_selector/7 -> TrnIgnOffDly_T_Rq/1  "<TrnIgnOffDly_T_Rq>"
  bus_selector/8 -> TrnPrkSys_D_Actl/1  "<TrnPrkSys_D_Actl>"
  bus_selector/9 -> TrnRng_D_Rq/1  "<TrnRng_D_Rq>"

== system test_mdl_NI/Subsystem/PCM/PowertrainData_1_Ox421 ==
  in_port : Inport
  AirCondFluidHi_P_Actl : Terminator
  CoolantFanStepAct : Terminator
  ECMMILRequest : Terminator
  EngIdlShutDown_D_Stat : Terminator
  EngIdlShutDwnTxt_D_Rq : Terminator
  FUEL_ALCOHOL_PERCNT : Terminator
  FohEng_D_Rq : Terminator
  OilPressureWarning : Terminator
  TrnTotLss_Tq_Est : Terminator
  TrnTotTq_Rt_Est : Terminator
  VehVLimActv_B_Actl : Terminator
  VehVLimStat_D_Actl : Terminator
  bus_selector : BusSelector  OutputSignals=AirCondFluidHi_P_Actl,CoolantFanStepAct,ECMMILRequest,EngIdlShutDown_D_Stat,EngIdlShutDwnTxt_D_Rq,FUEL_ALCOHOL_PERCNT,FohEng_D_Rq,OilPressureWarning,TrnTotLss_Tq_Est,TrnTotTq_Rt_Est,VehVLimActv_B_Actl,VehVLimStat_D_Actl
  wires:
  in_port/1 -> bus_selector/1  "PowertrainData_1_Ox421"
  bus_selector/1 -> AirCondFluidHi_P_Actl/1  "<AirCondFluidHi_P_Actl>"
  bus_selector/2 -> CoolantFanStepAct/1  "<CoolantFanStepAct>"
  bus_selector/3 -> ECMMILRequest/1  "<ECMMILRequest>"
  bus_selector/4 -> EngIdlShutDown_D_Stat/1  "<EngIdlShutDown_D_Stat>"
  bus_selector/5 -> EngIdlShutDwnTxt_D_Rq/1  "<EngIdlShutDwnTxt_D_Rq>"
  bus_selector/6 -> FUEL_ALCOHOL_PERCNT/1  "<FUEL_ALCOHOL_PERCNT>"
  bus_selector/7 -> FohEng_D_Rq/1  "<FohEng_D_Rq>"
  bus_selector/8 -> OilPressureWarning/1  "<OilPressureWarning>"
  bus_selector/9 -> TrnTotLss_Tq_Est/1  "<TrnTotLss_Tq_Est>"
  bus_selector/10 -> TrnTotTq_Rt_Est/1  "<TrnTotTq_Rt_Est>"
  bus_selector/11 -> VehVLimActv_B_Actl/1  "<VehVLimActv_B_Actl>"
  bus_selector/12 -> VehVLimStat_D_Actl/1  "<VehVLimStat_D_Actl>"

== system test_mdl_NI/Subsystem/PCM/PowertrainData_2_Ox42D ==
  in_port : Inport
  ApedPos_Pc_ActlDiag : Terminator
  EngAirIn_Te_Actl : Terminator
  EngClnt_Te_ActlDiag : Terminator
  EngLoad_Pc_CalcDiag : Terminator
  EngMsgTxt_D_Rq : Terminator
  GrllShtrPos_B_Falt : Terminator
  GrllShtrPos_D_Cmd : Terminator
  IsaOffst_D_Stat : Terminator
  ObdWarmUp_B_Complt : Terminator
  SlMde_D_RqDsply : Terminator
  SlMde_D_Stat : Terminator
  bus_selector : BusSelector  OutputSignals=ApedPos_Pc_ActlDiag,EngAirIn_Te_Actl,EngClnt_Te_ActlDiag,EngLoad_Pc_CalcDiag,EngMsgTxt_D_Rq,GrllShtrPos_B_Falt,GrllShtrPos_D_Cmd,IsaOffst_D_Stat,ObdWarmUp_B_Complt,SlMde_D_RqDsply,SlMde_D_Stat
  wires:
  in_port/1 -> bus_selector/1  "PowertrainData_2_Ox42D"
  bus_selector/1 -> ApedPos_Pc_ActlDiag/1  "<ApedPos_Pc_ActlDiag>"
  bus_selector/2 -> EngAirIn_Te_Actl/1  "<EngAirIn_Te_Actl>"
  bus_selector/3 -> EngClnt_Te_ActlDiag/1  "<EngClnt_Te_ActlDiag>"
  bus_selector/4 -> EngLoad_Pc_CalcDiag/1  "<EngLoad_Pc_CalcDiag>"
  bus_selector/5 -> EngMsgTxt_D_Rq/1  "<EngMsgTxt_D_Rq>"
  bus_selector/6 -> GrllShtrPos_B_Falt/1  "<GrllShtrPos_B_Falt>"
  bus_selector/7 -> GrllShtrPos_D_Cmd/1  "<GrllShtrPos_D_Cmd>"
  bus_selector/8 -> IsaOffst_D_Stat/1  "<IsaOffst_D_Stat>"
  bus_selector/9 -> ObdWarmUp_B_Complt/1  "<ObdWarmUp_B_Complt>"
  bus_selector/10 -> SlMde_D_RqDsply/1  "<SlMde_D_RqDsply>"
  bus_selector/11 -> SlMde_D_Stat/1  "<SlMde_D_Stat>"

== system test_mdl_NI/Subsystem/PCM/PowertrainData_3_Ox43E ==
  in_port : Inport
  BattULoChrg_U_Cmd : Terminator
  ElLoadCtl_D_Rq : Terminator
  EngMnfld_P_Actl : Terminator
  FuelPumpPwr_B_Rq : Terminator
  bus_selector : BusSelector  OutputSignals=BattULoChrg_U_Cmd,ElLoadCtl_D_Rq,EngMnfld_P_Actl,FuelPumpPwr_B_Rq
  wires:
  in_port/1 -> bus_selector/1  "PowertrainData_3_Ox43E"
  bus_selector/1 -> BattULoChrg_U_Cmd/1  "<BattULoChrg_U_Cmd>"
  bus_selector/2 -> ElLoadCtl_D_Rq/1  "<ElLoadCtl_D_Rq>"
  bus_selector/3 -> EngMnfld_P_Actl/1  "<EngMnfld_P_Actl>"
  bus_selector/4 -> FuelPumpPwr_B_Rq/1  "<FuelPumpPwr_B_Rq>"

== system test_mdl_NI/Subsystem/PCM/PowertrainData_6_Ox205 ==
  in_port : Inport
  BrkTot_Tq_RqFapLc : Terminator
  FapLc_B_Err : Terminator
  TrnAin_Pc_RqDrv : Terminator
  bus_selector : BusSelector  OutputSignals=BrkTot_Tq_RqFapLc,FapLc_B_Err,TrnAin_Pc_RqDrv
  wires:
  in_port/1 -> bus_selector/1  "PowertrainData_6_Ox205"
  bus_selector/1 -> BrkTot_Tq_RqFapLc/1  "<BrkTot_Tq_RqFapLc>"
  bus_selector/2 -> FapLc_B_Err/1  "<FapLc_B_Err>"
  bus_selector/3 -> TrnAin_Pc_RqDrv/1  "<TrnAin_Pc_RqDrv>"

== system test_mdl_NI/Subsystem/PCM/PowertrainData_7_Ox41F ==
  in_port : Inport
  EcoCochA_Pc_Dsply : Terminator
  EcoCochCrus_Pc_Dsply : Terminator
  EcoCochDecel_Pc_Dsply : Terminator
  EcoCochIdlFuel_Pc_Dsply : Terminator
  EcoCochInstNeg_B_Dsply : Terminator
  EcoCochInst_Pc_Dsply : Terminator
  EcoCochShif_Pc_Dsply : Terminator
  bus_selector : BusSelector  OutputSignals=EcoCochA_Pc_Dsply,EcoCochCrus_Pc_Dsply,EcoCochDecel_Pc_Dsply,EcoCochIdlFuel_Pc_Dsply,EcoCochInstNeg_B_Dsply,EcoCochInst_Pc_Dsply,EcoCochShif_Pc_Dsply
  wires:
  in_port/1 -> bus_selector/1  "PowertrainData_7_Ox41F"
  bus_selector/1 -> EcoCochA_Pc_Dsply/1  "<EcoCochA_Pc_Dsply>"
  bus_selector/2 -> EcoCochCrus_Pc_Dsply/1  "<EcoCochCrus_Pc_Dsply>"
  bus_selector/3 -> EcoCochDecel_Pc_Dsply/1  "<EcoCochDecel_Pc_Dsply>"
  bus_selector/4 -> EcoCochIdlFuel_Pc_Dsply/1  "<EcoCochIdlFuel_Pc_Dsply>"
  bus_selector/5 -> EcoCochInstNeg_B_Dsply/1  "<EcoCochInstNeg_B_Dsply>"
  bus_selector/6 -> EcoCochInst_Pc_Dsply/1  "<EcoCochInst_Pc_Dsply>"
  bus_selector/7 -> EcoCochShif_Pc_Dsply/1  "<EcoCochShif_Pc_Dsply>"

== system test_mdl_NI/Subsystem/PCM/PowertrainData_9_Ox44C ==
  in_port : Inport
  AutoTowActv_B_Stat : Terminator
  AutoTowAllw_D_StatMnu : Terminator
  EngExhMdeQuiet_D2_Stat : Terminator
  GrossTrainWeight_M_Est : Terminator
  HvacCmprLim_D_Stat : Terminator
  TrailCtlPt_B_Falt : Terminator
  Veh_V_DsplyTrailCtlSet : Terminator
  WakeAlarm1_B_Typ : Terminator
  WakeAlarm1_T_Rq : Terminator
  bus_selector : BusSelector  OutputSignals=AutoTowActv_B_Stat,AutoTowAllw_D_StatMnu,EngExhMdeQuiet_D2_Stat,GrossTrainWeight_M_Est,HvacCmprLim_D_Stat,TrailCtlPt_B_Falt,Veh_V_DsplyTrailCtlSet,WakeAlarm1_B_Typ,WakeAlarm1_T_Rq
  wires:
  in_port/1 -> bus_selector/1  "PowertrainData_9_Ox44C"
  bus_selector/1 -> AutoTowActv_B_Stat/1  "<AutoTowActv_B_Stat>"
  bus_selector/2 -> AutoTowAllw_D_StatMnu/1  "<AutoTowAllw_D_StatMnu>"
  bus_selector/3 -> EngExhMdeQuiet_D2_Stat/1  "<EngExhMdeQuiet_D2_Stat>"
  bus_selector/4 -> GrossTrainWeight_M_Est/1  "<GrossTrainWeight_M_Est>"
  bus_selector/5 -> HvacCmprLim_D_Stat/1  "<HvacCmprLim_D_Stat>"
  bus_selector/6 -> TrailCtlPt_B_Falt/1  "<TrailCtlPt_B_Falt>"
  bus_selector/7 -> Veh_V_DsplyTrailCtlSet/1  "<Veh_V_DsplyTrailCtlSet>"
  bus_selector/8 -> WakeAlarm1_B_Typ/1  "<WakeAlarm1_B_Typ>"
  bus_selector/9 -> WakeAlarm1_T_Rq/1  "<WakeAlarm1_T_Rq>"

== system test_mdl_NI/Subsystem/PCM/Powertrain_Data_4_Ox424 ==
  in_port : Inport
  BpedDrvMsgTxt_B_Dsply : Terminator
  FuelLvlWarn_D_ActlEng : Terminator
  FuelLvl_Pc_DsplyEng : Terminator
  FuelRange_L_DsplyEng : Terminator
  RearDiffOilTeWarn_B_Rq : Terminator
  RearDiffOil_Te_Actl : Terminator
  SelDrvMdePt_D_Stat : Terminator
  bus_selector : BusSelector  OutputSignals=BpedDrvMsgTxt_B_Dsply,FuelLvlWarn_D_ActlEng,FuelLvl_Pc_DsplyEng,FuelRange_L_DsplyEng,RearDiffOilTeWarn_B_Rq,RearDiffOil_Te_Actl,SelDrvMdePt_D_Stat
  wires:
  in_port/1 -> bus_selector/1  "Powertrain_Data_4_Ox424"
  bus_selector/1 -> BpedDrvMsgTxt_B_Dsply/1  "<BpedDrvMsgTxt_B_Dsply>"
  bus_selector/2 -> FuelLvlWarn_D_ActlEng/1  "<FuelLvlWarn_D_ActlEng>"
  bus_selector/3 -> FuelLvl_Pc_DsplyEng/1  "<FuelLvl_Pc_DsplyEng>"
  bus_selector/4 -> FuelRange_L_DsplyEng/1  "<FuelRange_L_DsplyEng>"
  bus_selector/5 -> RearDiffOilTeWarn_B_Rq/1  "<RearDiffOilTeWarn_B_Rq>"
  bus_selector/6 -> RearDiffOil_Te_Actl/1  "<RearDiffOil_Te_Actl>"
  bus_selector/7 -> SelDrvMdePt_D_Stat/1  "<SelDrvMdePt_D_Stat>"

== system test_mdl_NI/Subsystem/PCM/Powertrain_Data_5_Ox43F ==
  in_port : Inport
  AdasLcObtclAbrt_B_Stat : Terminator
  AirDamPos_D_Stat : Terminator
  BattRgenLoChrg_D_RqEng : Terminator
  BattRgenLoDChrg_D_RqEng : Terminator
  FapLcActv_B_Stat : Terminator
  FapLcInhbt_B_Rq : Terminator
  FapLcMaxGrdAbrt_B_Stat : Terminator
  FapLcMaxGrdInhbt_B_Stat : Terminator
  FapLcObstcl_B_Stat : Terminator
  FapLcPrchgBrk_B_Rq : Terminator
  FapLcStopHold_B_Rq : Terminator
  bus_selector : BusSelector  OutputSignals=AdasLcObtclAbrt_B_Stat,AirDamPos_D_Stat,BattRgenLoChrg_D_RqEng,BattRgenLoDChrg_D_RqEng,FapLcActv_B_Stat,FapLcInhbt_B_Rq,FapLcMaxGrdAbrt_B_Stat,FapLcMaxGrdInhbt_B_Stat,FapLcObstcl_B_Stat,FapLcPrchgBrk_B_Rq,FapLcStopHold_B_Rq
  wires:
  in_port/1 -> bus_selector/1  "Powertrain_Data_5_Ox43F"
  bus_selector/1 -> AdasLcObtclAbrt_B_Stat/1  "<AdasLcObtclAbrt_B_Stat>"
  bus_selector/2 -> AirDamPos_D_Stat/1  "<AirDamPos_D_Stat>"
  bus_selector/3 -> BattRgenLoChrg_D_RqEng/1  "<BattRgenLoChrg_D_RqEng>"
  bus_selector/4 -> BattRgenLoDChrg_D_RqEng/1  "<BattRgenLoDChrg_D_RqEng>"
  bus_selector/5 -> FapLcActv_B_Stat/1  "<FapLcActv_B_Stat>"
  bus_selector/6 -> FapLcInhbt_B_Rq/1  "<FapLcInhbt_B_Rq>"
  bus_selector/7 -> FapLcMaxGrdAbrt_B_Stat/1  "<FapLcMaxGrdAbrt_B_Stat>"
  bus_selector/8 -> FapLcMaxGrdInhbt_B_Stat/1  "<FapLcMaxGrdInhbt_B_Stat>"
  bus_selector/9 -> FapLcObstcl_B_Stat/1  "<FapLcObstcl_B_Stat>"
  bus_selector/10 -> FapLcPrchgBrk_B_Rq/1  "<FapLcPrchgBrk_B_Rq>"
  bus_selector/11 -> FapLcStopHold_B_Rq/1  "<FapLcStopHold_B_Rq>"

== system test_mdl_NI/Subsystem/PCM/Stop_Start_Ox166 ==
  in_port : Inport
  AutoStopPtDelta_I_Est : Terminator
  HiElPwInhbt_B_Stat : Terminator
  OdoTripVerify_L_Actl : Terminator
  StopStrtDrvMde_D_Indic : Terminator
  StopStrtIODTxt_D_Rq : Terminator
  StopStrtMsgTxt_D_Rq : Terminator
  StopStrtStdby_D_Indic : Terminator
  bus_selector : BusSelector  OutputSignals=AutoStopPtDelta_I_Est,HiElPwInhbt_B_Stat,OdoTripVerify_L_Actl,StopStrtDrvMde_D_Indic,StopStrtIODTxt_D_Rq,StopStrtMsgTxt_D_Rq,StopStrtStdby_D_Indic
  wires:
  in_port/1 -> bus_selector/1  "Stop_Start_Ox166"
  bus_selector/1 -> AutoStopPtDelta_I_Est/1  "<AutoStopPtDelta_I_Est>"
  bus_selector/2 -> HiElPwInhbt_B_Stat/1  "<HiElPwInhbt_B_Stat>"
  bus_selector/3 -> OdoTripVerify_L_Actl/1  "<OdoTripVerify_L_Actl>"
  bus_selector/4 -> StopStrtDrvMde_D_Indic/1  "<StopStrtDrvMde_D_Indic>"
  bus_selector/5 -> StopStrtIODTxt_D_Rq/1  "<StopStrtIODTxt_D_Rq>"
  bus_selector/6 -> StopStrtMsgTxt_D_Rq/1  "<StopStrtMsgTxt_D_Rq>"
  bus_selector/7 -> StopStrtStdby_D_Indic/1  "<StopStrtStdby_D_Indic>"

== system test_mdl_NI/Subsystem/PCM/TesterPhysicalResPCM_Ox7E8 ==
  in_port : Inport
  TesterPhysicalResPCM : Terminator
  bus_selector : BusSelector  OutputSignals=TesterPhysicalResPCM
  wires:
  in_port/1 -> bus_selector/1  "TesterPhysicalResPCM_Ox7E8"
  bus_selector/1 -> TesterPhysicalResPCM/1  "<TesterPhysicalResPCM>"

== system test_mdl_NI/Subsystem/PCM/TorqueDataEngFlags_Ox200 ==
  in_port : Inport
  PrplWhlTotTqRq_No_Cnt : Terminator
  PrplWhlTotTqRq_No_Cs : Terminator
  PrplWhlTot_Tq_LimMn : Terminator
  PrplWhlTot_Tq_Rq : Terminator
  PtDrvMde_D_Stat : Terminator
  bus_selector : BusSelector  OutputSignals=PrplWhlTotTqRq_No_Cnt,PrplWhlTotTqRq_No_Cs,PrplWhlTot_Tq_LimMn,PrplWhlTot_Tq_Rq,PtDrvMde_D_Stat
  wires:
  in_port/1 -> bus_selector/1  "TorqueDataEngFlags_Ox200"
  bus_selector/1 -> PrplWhlTotTqRq_No_Cnt/1  "<PrplWhlTotTqRq_No_Cnt>"
  bus_selector/2 -> PrplWhlTotTqRq_No_Cs/1  "<PrplWhlTotTqRq_No_Cs>"
  bus_selector/3 -> PrplWhlTot_Tq_LimMn/1  "<PrplWhlTot_Tq_LimMn>"
  bus_selector/4 -> PrplWhlTot_Tq_Rq/1  "<PrplWhlTot_Tq_Rq>"
  bus_selector/5 -> PtDrvMde_D_Stat/1  "<PtDrvMde_D_Stat>"

== system test_mdl_NI/Subsystem/PCM/TransGearData_Ox230 ==
  in_port : Inport
  GboxOil_Te_Actl : Terminator
  GearLvrPos_D_Actl : Terminator
  SelDrvMdeSwtch_D_Stat3 : Terminator
  TrnShifActv_B_Actl : Terminator
  TrnSrvcRqd_B_Rq : Terminator
  bus_selector : BusSelector  OutputSignals=GboxOil_Te_Actl,GearLvrPos_D_Actl,SelDrvMdeSwtch_D_Stat3,TrnShifActv_B_Actl,TrnSrvcRqd_B_Rq
  wires:
  in_port/1 -> bus_selector/1  "TransGearData_Ox230"
  bus_selector/1 -> GboxOil_Te_Actl/1  "<GboxOil_Te_Actl>"
  bus_selector/2 -> GearLvrPos_D_Actl/1  "<GearLvrPos_D_Actl>"
  bus_selector/3 -> SelDrvMdeSwtch_D_Stat3/1  "<SelDrvMdeSwtch_D_Stat3>"
  bus_selector/4 -> TrnShifActv_B_Actl/1  "<TrnShifActv_B_Actl>"
  bus_selector/5 -> TrnSrvcRqd_B_Rq/1  "<TrnSrvcRqd_B_Rq>"

== system test_mdl_NI/Subsystem/PCM/VehicleOperatingModes_Ox167 ==
  in_port : Inport
  ElPw_D_Stat : Terminator
  ElPw_D_StatStrtStop : Terminator
  Eng_D_Stat : Terminator
  PlgActvArb_B_Actl : Terminator
  PrplWhlRgenMn_Tq_Actl : Terminator
  PrplWhlTot2_Tq_Actl : Terminator
  PwPckTq_D_Stat : Terminator
  TrnAinTq_D_Qf : Terminator
  TrnAin_Tq_Actl : Terminator
  bus_selector : BusSelector  OutputSignals=ElPw_D_Stat,ElPw_D_StatStrtStop,Eng_D_Stat,PlgActvArb_B_Actl,PrplWhlRgenMn_Tq_Actl,PrplWhlTot2_Tq_Actl,PwPckTq_D_Stat,TrnAinTq_D_Qf,TrnAin_Tq_Actl
  wires:
  in_port/1 -> bus_selector/1  "VehicleOperatingModes_Ox167"
  bus_selector/1 -> ElPw_D_Stat/1  "<ElPw_D_Stat>"
  bus_selector/2 -> ElPw_D_StatStrtStop/1  "<ElPw_D_StatStrtStop>"
  bus_selector/3 -> Eng_D_Stat/1  "<Eng_D_Stat>"
  bus_selector/4 -> PlgActvArb_B_Actl/1  "<PlgActvArb_B_Actl>"
  bus_selector/5 -> PrplWhlRgenMn_Tq_Actl/1  "<PrplWhlRgenMn_Tq_Actl>"
  bus_selector/6 -> PrplWhlTot2_Tq_Actl/1  "<PrplWhlTot2_Tq_Actl>"
  bus_selector/7 -> PwPckTq_D_Stat/1  "<PwPckTq_D_Stat>"
  bus_selector/8 -> TrnAinTq_D_Qf/1  "<TrnAinTq_D_Qf>"
  bus_selector/9 -> TrnAin_Tq_Actl/1  "<TrnAin_Tq_Actl>"

== system test_mdl_NI/Subsystem/PCM_HEV/Cluster_HEV_Data10_FD1_Ox471 ==
  in_port : Inport
  RngPerChrgAvg_L_Dsply : Terminator
  bus_selector : BusSelector  OutputSignals=RngPerChrgAvg_L_Dsply
  wires:
  in_port/1 -> bus_selector/1  "Cluster_HEV_Data10_FD1_Ox471"
  bus_selector/1 -> RngPerChrgAvg_L_Dsply/1  "<RngPerChrgAvg_L_Dsply>"

== system test_mdl_NI/Subsystem/PCM_HEV/Cluster_HEV_Data1_FD1_Ox312 ==
  in_port : Inport
  ChrgStat_D_Dsply : Terminator
  RgenTrip_L_Dsply : Terminator
  RgenTrip_Pc_Dsply : Terminator
  bus_selector : BusSelector  OutputSignals=ChrgStat_D_Dsply,RgenTrip_L_Dsply,RgenTrip_Pc_Dsply
  wires:
  in_port/1 -> bus_selector/1  "Cluster_HEV_Data1_FD1_Ox312"
  bus_selector/1 -> ChrgStat_D_Dsply/1  "<ChrgStat_D_Dsply>"
  bus_selector/2 -> RgenTrip_L_Dsply/1  "<RgenTrip_L_Dsply>"
  bus_selector/3 -> RgenTrip_Pc_Dsply/1  "<RgenTrip_Pc_Dsply>"

== system test_mdl_NI/Subsystem/PCM_HEV/Cluster_HEV_Data2_Ox365 ==
  in_port : Inport
  EffWhlLvl2_Pc_Dsply : Terminator
  EffWhlThresOn_B_Dsply : Terminator
  EffWhlThres_Pc_Dsply : Terminator
  EngActv_B_Dsply : Terminator
  EngOnMsg1_D_Dsply : Terminator
  EngOnMsg2_D_Dsply : Terminator
  EngPwLvl_Pc_Dsply : Terminator
  FuelMaintMde_D_Dsply : Terminator
  PwrFlowTxt_D_Dsply : Terminator
  bus_selector : BusSelector  OutputSignals=EffWhlLvl2_Pc_Dsply,EffWhlThresOn_B_Dsply,EffWhlThres_Pc_Dsply,EngActv_B_Dsply,EngOnMsg1_D_Dsply,EngOnMsg2_D_Dsply,EngPwLvl_Pc_Dsply,FuelMaintMde_D_Dsply,PwrFlowTxt_D_Dsply
  wires:
  in_port/1 -> bus_selector/1  "Cluster_HEV_Data2_Ox365"
  bus_selector/1 -> EffWhlLvl2_Pc_Dsply/1  "<EffWhlLvl2_Pc_Dsply>"
  bus_selector/2 -> EffWhlThresOn_B_Dsply/1  "<EffWhlThresOn_B_Dsply>"
  bus_selector/3 -> EffWhlThres_Pc_Dsply/1  "<EffWhlThres_Pc_Dsply>"
  bus_selector/4 -> EngActv_B_Dsply/1  "<EngActv_B_Dsply>"
  bus_selector/5 -> EngOnMsg1_D_Dsply/1  "<EngOnMsg1_D_Dsply>"
  bus_selector/6 -> EngOnMsg2_D_Dsply/1  "<EngOnMsg2_D_Dsply>"
  bus_selector/7 -> EngPwLvl_Pc_Dsply/1  "<EngPwLvl_Pc_Dsply>"
  bus_selector/8 -> FuelMaintMde_D_Dsply/1  "<FuelMaintMde_D_Dsply>"
  bus_selector/9 -> PwrFlowTxt_D_Dsply/1  "<PwrFlowTxt_D_Dsply>"

== system test_mdl_NI/Subsystem/PCM_HEV/Cluster_HEV_Data3_FD1_Ox366 ==
  in_port : Inport
  EffRgenThres_Pc_Dsply : Terminator
  EngMdeMsgTxt_D_Rq : Terminator
  RngPerChrgInst_L_Dsply : Terminator
  bus_selector : BusSelector  OutputSignals=EffRgenThres_Pc_Dsply,EngMdeMsgTxt_D_Rq,RngPerChrgInst_L_Dsply
  wires:
  in_port/1 -> bus_selector/1  "Cluster_HEV_Data3_FD1_Ox366"
  bus_selector/1 -> EffRgenThres_Pc_Dsply/1  "<EffRgenThres_Pc_Dsply>"
  bus_selector/2 -> EngMdeMsgTxt_D_Rq/1  "<EngMdeMsgTxt_D_Rq>"
  bus_selector/3 -> RngPerChrgInst_L_Dsply/1  "<RngPerChrgInst_L_Dsply>"

== system test_mdl_NI/Subsystem/PCM_HEV/Cluster_HEV_Data5_Ox368 ==
  in_port : Inport
  HybMdeStat_D_Dsply : Terminator
  PlgActvArb_B_Dsply : Terminator
  bus_selector : BusSelector  OutputSignals=HybMdeStat_D_Dsply,PlgActvArb_B_Dsply
  wires:
  in_port/1 -> bus_selector/1  "Cluster_HEV_Data5_Ox368"
  bus_selector/1 -> HybMdeStat_D_Dsply/1  "<HybMdeStat_D_Dsply>"
  bus_selector/2 -> PlgActvArb_B_Dsply/1  "<PlgActvArb_B_Dsply>"

== system test_mdl_NI/Subsystem/PCM_HEV/DCACA_Data4_Ox36E ==
  in_port : Inport
  DcacElPw_D_Stat : Terminator
  DcacEngOnMsgTxt_D_Rq : Terminator
  DcacFaltMsgTxt_D_Rq : Terminator
  DcacGfciTest_B_Rq : Terminator
  DcacHw_D_Confg : Terminator
  DcacLedCtl_D_Rq : Terminator
  DcacLoFuelMsgTxt_D_Rq : Terminator
  DcacOn_B_Rq : Terminator
  DcacOut1_Pw_Dsply : Terminator
  DcacOut2_Pw_Dsply : Terminator
  DcacOut_Pw_DsplyMx : Terminator
  DcacSys_B_Falt : Terminator
  PwBedPnlEnbl_B_Rq : Terminator
  bus_selector : BusSelector  OutputSignals=DcacElPw_D_Stat,DcacEngOnMsgTxt_D_Rq,DcacFaltMsgTxt_D_Rq,DcacGfciTest_B_Rq,DcacHw_D_Confg,DcacLedCtl_D_Rq,DcacLoFuelMsgTxt_D_Rq,DcacOn_B_Rq,DcacOut1_Pw_Dsply,DcacOut2_Pw_Dsply,DcacOut_Pw_DsplyMx,DcacSys_B_Falt,PwBedPnlEnbl_B_Rq
  wires:
  in_port/1 -> bus_selector/1  "DCACA_Data4_Ox36E"
  bus_selector/1 -> DcacElPw_D_Stat/1  "<DcacElPw_D_Stat>"
  bus_selector/2 -> DcacEngOnMsgTxt_D_Rq/1  "<DcacEngOnMsgTxt_D_Rq>"
  bus_selector/3 -> DcacFaltMsgTxt_D_Rq/1  "<DcacFaltMsgTxt_D_Rq>"
  bus_selector/4 -> DcacGfciTest_B_Rq/1  "<DcacGfciTest_B_Rq>"
  bus_selector/5 -> DcacHw_D_Confg/1  "<DcacHw_D_Confg>"
  bus_selector/6 -> DcacLedCtl_D_Rq/1  "<DcacLedCtl_D_Rq>"
  bus_selector/7 -> DcacLoFuelMsgTxt_D_Rq/1  "<DcacLoFuelMsgTxt_D_Rq>"
  bus_selector/8 -> DcacOn_B_Rq/1  "<DcacOn_B_Rq>"
  bus_selector/9 -> DcacOut1_Pw_Dsply/1  "<DcacOut1_Pw_Dsply>"
  bus_selector/10 -> DcacOut2_Pw_Dsply/1  "<DcacOut2_Pw_Dsply>"
  bus_selector/11 -> DcacOut_Pw_DsplyMx/1  "<DcacOut_Pw_DsplyMx>"
  bus_selector/12 -> DcacSys_B_Falt/1  "<DcacSys_B_Falt>"
  bus_selector/13 -> PwBedPnlEnbl_B_Rq/1  "<PwBedPnlEnbl_B_Rq>"
